simulink model "DR18E_Testpult"  (R2017a)
settings: Solver=ode1  StartTime=0.0  StopTime=Inf  FixedStep=0.001  RelTol=1e-3
PostLoadFcn:
  | , if any(exist('dsrtsu_mdlpostloadfcn', 'file') == [2, 3, 6]), try dsrtsu_mdlpostloadfcn('Execute', bdroot); catch fprintf('Error in PostLoadFcn (dsrtsu_mdlpostloadfcn) for model "%s":\n %s\n', bdroot, lasterr); end, end,
model workspace: external: MATLAB File C:\Users\DeltaRacing\Documents\dSPACE\MABX_DR18E\Model\DR18E_MABX_Parameter.m (data not in the file)
values from neighbouring files (symbols this model uses):
  am = 1/Ts    (= 1)    [DR18E_MABX_Parameter.m]
  bm = K/Ts    (= 0.05)    [DR18E_MABX_Parameter.m]
  cf = 41350    [DR18E_MABX_Parameter.m]
  cr = 41350    [DR18E_MABX_Parameter.m]
  Derating_HV_Battery_Kapa = 1    [DR18E_MABX_Parameter.m]
  Derating_Start_km = 16    [DR18E_MABX_Parameter.m]
  Drive_Mode = 0    [DR18E_MABX_Parameter.m]
  g = 1    [DR18E_MABX_Parameter.m]
  Gas_Modus = 2    [DR18E_MABX_Parameter.m]
  HV_Power_max = 80    [DR18E_MABX_Parameter.m]
  i_Getriebe = 3.3    [DR18E_MABX_Parameter.m]
  i_Lenkgetriebe = 4.32    [DR18E_MABX_Parameter.m]
  K_SET = 1    [DR18E_MABX_Parameter.m]
  Kapazitaet_HV_Battery_kWh = 6.6    [DR18E_MABX_Parameter.m]
  KW_T_Soll = 37    [DR18E_MABX_Parameter.m]
  lf = 1.2    [DR18E_MABX_Parameter.m]
  lr = 1.15    [DR18E_MABX_Parameter.m]
  m = 310    [DR18E_MABX_Parameter.m]
  M_max = 150    [DR18E_MABX_Parameter.m]
  Power_Limit_onoff = 0    [DR18E_MABX_Parameter.m]
  Reifenradius = 0.2351    [DR18E_MABX_Parameter.m]
  Strecke_Endu_km = 22    [DR18E_MABX_Parameter.m]
  TC_Decr_Gas = 0.00005    (= 5e-05)    [DR18E_MABX_Parameter.m]
  TC_Derivative = 0.4    [DR18E_MABX_Parameter.m]
  TC_Incr_Gas = 0.005    [DR18E_MABX_Parameter.m]
  TC_On = 0    [DR18E_MABX_Parameter.m]
  TC_Relay_Off = 0.065    [DR18E_MABX_Parameter.m]
  TC_Relay_On = 0.07    [DR18E_MABX_Parameter.m]
  TV_Mode = 2    [DR18E_MABX_Parameter.m]
  TV_On = 0    [DR18E_MABX_Parameter.m]
  TV_Override = 1    [DR18E_MABX_Parameter.m]
  y = 0.8    [DR18E_MABX_Parameter.m]
undefined symbols (not defined in the file or in its folder): D, DiscIntNeverNeededParam, I, K_OL, P
libraries: simulink x288, rtican x105, rtiusbflightreclib x40, rti1401lib_dio_type3 x10, simulink_extras x10, rti1401lib_adc_type4 x8, rti1401lib_II_base x7
(part 19 of 28)

== system DR18E_Testpult/Verarbeitung/Temperaturregelung1/ModeSelect1 ==
  Man/Aut Pulse : Inport
  Value Man : Inport  Port=2
  Value Aut : Inport  Port=3
  Constant : Constant  OutDataTypeStr=Inherit: Inherit via back propagation
  Data Type Conversion : DataTypeConversion  OutDataTypeStr=boolean
  J-K Flip-Flop : simulink_extras/Flip Flops/J-K Flip-Flop  initial_condition=0
      settings: SourceProductName=Simulink
  Switch : Switch  Criteria=u2 > Threshold
  Value : Outport
  wires:
  Value Man/1 -> Switch/1
  Value Aut/1 -> Switch/3
  Switch/1 -> Value/1
  Constant/1 -> J-K Flip-Flop/3, J-K Flip-Flop/1
  Man/Aut Pulse/1 -> Data Type Conversion/1
  J-K Flip-Flop/1 -> Switch/2  "Man/!Aut"
  Data Type Conversion/1 -> J-K Flip-Flop/2

== system DR18E_Testpult/Verarbeitung/Temperaturregelung1/ModeSelect2 ==
  Man/Aut Pulse : Inport
  Value Man : Inport  Port=2
  Value Aut : Inport  Port=3
  Constant : Constant  OutDataTypeStr=Inherit: Inherit via back propagation
  Data Type Conversion : DataTypeConversion  OutDataTypeStr=boolean
  J-K Flip-Flop : simulink_extras/Flip Flops/J-K Flip-Flop  initial_condition=0
      settings: SourceProductName=Simulink
  Switch : Switch  Criteria=u2 > Threshold
  Value : Outport
  wires:
  Value Man/1 -> Switch/1
  Value Aut/1 -> Switch/3
  Switch/1 -> Value/1
  Constant/1 -> J-K Flip-Flop/3, J-K Flip-Flop/1
  Man/Aut Pulse/1 -> Data Type Conversion/1
  J-K Flip-Flop/1 -> Switch/2  "Man/!Aut"
  Data Type Conversion/1 -> J-K Flip-Flop/2

== system DR18E_Testpult/Verarbeitung/Temperaturregelung1/PT1 Discrete ==
  u : Inport
  K : Inport  Port=2
  T : Inport  Port=3
  Memory : Memory
  Product : Product
  Product1 : Product
  Subsystem : Subsystem
  Sum : Sum  Inputs=|+-
  Sum1 : Sum  Inputs=|++
  y : Outport
  wires:
  K/1 -> Product/1
  Subsystem/1(T*) -> Product1/1
  u/1 -> Product/2
  Sum/1 -> Product1/2
  Product1/1 -> Sum1/1
  Memory/1 -> Sum1/2, Sum/2
  Sum1/1 -> y/1, Memory/1
  Product/1 -> Sum/1
  T/1 -> Subsystem/1(T)

== system DR18E_Testpult/Verarbeitung/Temperaturregelung1/PT1 Discrete1 ==
  u : Inport
  K : Inport  Port=2
  T : Inport  Port=3
  Memory : Memory
  Product : Product
  Product1 : Product
  Subsystem : Subsystem
  Sum : Sum  Inputs=|+-
  Sum1 : Sum  Inputs=|++
  y : Outport
  wires:
  K/1 -> Product/1
  Subsystem/1(T*) -> Product1/1
  u/1 -> Product/2
  Sum/1 -> Product1/2
  Product1/1 -> Sum1/1
  Memory/1 -> Sum1/2, Sum/2
  Sum1/1 -> y/1, Memory/1
  Product/1 -> Sum/1
  T/1 -> Subsystem/1(T)

== system DR18E_Testpult/Verarbeitung/Umrichter Init Config/Umrichter 1 Init Config ==
  note: TX-Register
  note: TX-Intervallzeit in ms
  Bus Creator : BusCreator  Inputs=8
  Bus Creator1 : BusCreator  Inputs=8
  TXReg1 : Constant  Value=hex2dec('30')  OutDataTypeStr=uint16
  TXReg2 : Constant  Value=hex2dec('27')  OutDataTypeStr=uint16
  TXReg3 : Constant  Value=hex2dec('49')  OutDataTypeStr=uint16
  TXReg4 : Constant  Value=hex2dec('90')  OutDataTypeStr=uint16
  TXReg5 : Constant  Value=hex2dec('40')  OutDataTypeStr=uint16
  TXReg6 : Constant  Value=hex2dec('8F')  OutDataTypeStr=uint16
  TXReg7 : Constant  Value=hex2dec('EB')  OutDataTypeStr=uint16
  TXReg8 : Constant  Value=hex2dec('4A')  OutDataTypeStr=uint16
  TXZeit1 : Constant  Value=127  OutDataTypeStr=uint16
  TXZeit2 : Constant  Value=129  OutDataTypeStr=uint16
  TXZeit3 : Constant  Value=254  OutDataTypeStr=uint16
  TXZeit4 : Constant  Value=113  OutDataTypeStr=uint16
  TXZeit5 : Constant  Value=105  OutDataTypeStr=uint16
  TXZeit6 : Constant  Value=131  OutDataTypeStr=uint16
  TXZeit7 : Constant  Value=254  OutDataTypeStr=uint16
  TXZeit8 : Constant  Value=254  OutDataTypeStr=uint16
  tag scope: U1config_TXRegister=global, U1config_TXZeiten=global
  wires:
  Bus Creator/1 -> [U1config_TXRegister]
  TXReg1/1 -> Bus Creator/1  "Drehzahl Istwert"
  TXReg2/1 -> Bus Creator/2  "Drehmoment Istwert"
  TXReg3/1 -> Bus Creator/3  "Motortemp"
  TXReg4/1 -> Bus Creator/4  "DrehmomentSollwert"
  TXReg5/1 -> Bus Creator/5  "Statusmeldung"
  TXReg6/1 -> Bus Creator/6  "Errormeldung"
  TXReg7/1 -> Bus Creator/7  "U_DC"
  TXReg8/1 -> Bus Creator/8  "InverterTemp"
  Bus Creator1/1 -> [U1config_TXZeiten]
  TXZeit1/1 -> Bus Creator1/1
  TXZeit2/1 -> Bus Creator1/2
  TXZeit3/1 -> Bus Creator1/3
  TXZeit4/1 -> Bus Creator1/4
  TXZeit5/1 -> Bus Creator1/5
  TXZeit6/1 -> Bus Creator1/6
  TXZeit7/1 -> Bus Creator1/7
  TXZeit8/1 -> Bus Creator1/8

== system DR18E_Testpult/Verarbeitung/Umrichter Init Config/Umrichter 2 Init Config ==
  note: TX-Register
  note: TX-Intervallzeit in ms
  Bus Creator : BusCreator  Inputs=8
  Bus Creator1 : BusCreator  Inputs=8
  TXReg1 : Constant  Value=hex2dec('30')  OutDataTypeStr=uint16
  TXReg2 : Constant  Value=hex2dec('27')  OutDataTypeStr=uint16
  TXReg3 : Constant  Value=hex2dec('49')  OutDataTypeStr=uint16
  TXReg4 : Constant  Value=hex2dec('90')  OutDataTypeStr=uint16
  TXReg5 : Constant  Value=hex2dec('40')  OutDataTypeStr=uint16
  TXReg6 : Constant  Value=hex2dec('8F')  OutDataTypeStr=uint16
  TXReg7 : Constant  Value=hex2dec('EB')  OutDataTypeStr=uint16
  TXReg8 : Constant  Value=hex2dec('4A')  OutDataTypeStr=uint16
  TXZeit1 : Constant  Value=127  OutDataTypeStr=uint16
  TXZeit2 : Constant  Value=134  OutDataTypeStr=uint16
  TXZeit3 : Constant  Value=254  OutDataTypeStr=uint16
  TXZeit4 : Constant  Value=109  OutDataTypeStr=uint16
  TXZeit5 : Constant  Value=131  OutDataTypeStr=uint16
  TXZeit6 : Constant  Value=103  OutDataTypeStr=uint16
  TXZeit7 : Constant  Value=254  OutDataTypeStr=uint16
  TXZeit8 : Constant  Value=254  OutDataTypeStr=uint16
  tag scope: U2config_TXRegister=global, U2config_TXZeiten=global
  wires:
  Bus Creator/1 -> [U2config_TXRegister]
  TXReg1/1 -> Bus Creator/1  "Drehzahl Istwert"
  TXReg2/1 -> Bus Creator/2  "Drehmoment Istwert"
  TXReg3/1 -> Bus Creator/3  "Motortemp"
  TXReg4/1 -> Bus Creator/4  "DrehmomentSollwert"
  TXReg5/1 -> Bus Creator/5  "Statusmeldung"
  TXReg6/1 -> Bus Creator/6  "Errormeldung"
  TXReg7/1 -> Bus Creator/7  "U_DC"
  TXReg8/1 -> Bus Creator/8  "InverterTemp"
  Bus Creator1/1 -> [U2config_TXZeiten]
  TXZeit1/1 -> Bus Creator1/1
  TXZeit2/1 -> Bus Creator1/2
  TXZeit3/1 -> Bus Creator1/3
  TXZeit4/1 -> Bus Creator1/4
  TXZeit5/1 -> Bus Creator1/5
  TXZeit6/1 -> Bus Creator1/6
  TXZeit7/1 -> Bus Creator1/7
  TXZeit8/1 -> Bus Creator1/8

== system DR18E_Testpult/Verarbeitung/Vehicle State Machine/FlightRecorder ==
  In1 : Inport
  Data Type Conversion : DataTypeConversion
  Gain : Gain
  USB_FLIGHT_REC_BL1 : rtiusbflightreclib/USB_FLIGHT_REC_BL1  VarName=State  DataType=Single  SampleTime=-1  TLCFileName=rtiusbflightrecwrite  Reserved1=[]  Reserved2=[]  Reserved3=[]  Reserved4=[]  DSProperties=struct('RTI',struct('Version',uint32(3),'BlockType',struct('isSLSource',uint8(0),'isSLSink',uint8(1),'isHWSource',uint8(0),'isHWSink',uint8(0),'isSetup',uint8(0),'isInline',uint8(1),'isNonInline',uint8(0),'isInterrupt',uint8(0),'isChannelwise',uint8(0)),'IOBoardType',{{'DSUSB','FLIGHTREC'}},'UnitType','FLIGHTREC','Identifier','WRITE','DialogType','SL','BlockSet','RTIUSBFLIGHTREC','SlaveProcessor','NONE'))  RTIBlockInterface=struct('InputPortsActive',1,'InputPortsWidth',int32(1),'InputPortsDataType',{{'SS_SINGLE'}},'BlockDisplay',{{['Write to\nUSB Flight Recorder'],'center'}},'IconTransparency','off','InitLevel',3,'BlockName',struct('Token',{{'USB_FLIGHT_REC_BL1'}}),'MaskDescription',['Write input to the Flight Recorder. Recorded data can be referenced by the specified variable.'],'SampleTime',{{-1}})  RTIBlockParameters=struct('VarName',{{'State','OFF',[]}},'DataType',{{'Single','OFF',[]}},'SampleTime',{{-1,'OFF',[]}},'TLCFileName',{{'rtiusbflightrecwrite','OFF',[]}})  RTISFcnParameters=struct('VarName','char','DataType','char','SampleTime','double','TLCFileName','char')  RTIBlockParaDefault=struct('VarName','Var1','DataType','Single','SampleTime',-1,'TLCFileName','rtiusbflightrecwrite')
      settings: SourceProductName=dSPACE RTI USB Flight Rec Blockset
  wires:
  Data Type Conversion/1 -> USB_FLIGHT_REC_BL1/1
  In1/1 -> Gain/1
  Gain/1 -> Data Type Conversion/1

== system DR18E_Testpult/Verarbeitung/Vehicle State Machine/FlightRecorder1 ==
  In1 : Inport
  Data Type Conversion : DataTypeConversion
  Gain : Gain
  USB_FLIGHT_REC_BL1 : rtiusbflightreclib/USB_FLIGHT_REC_BL1  VarName=ErrorNo  DataType=Single  SampleTime=-1  TLCFileName=rtiusbflightrecwrite  Reserved1=[]  Reserved2=[]  Reserved3=[]  Reserved4=[]  DSProperties=struct('RTI',struct('Version',uint32(3),'BlockType',struct('isSLSource',uint8(0),'isSLSink',uint8(1),'isHWSource',uint8(0),'isHWSink',uint8(0),'isSetup',uint8(0),'isInline',uint8(1),'isNonInline',uint8(0),'isInterrupt',uint8(0),'isChannelwise',uint8(0)),'IOBoardType',{{'DSUSB','FLIGHTREC'}},'UnitType','FLIGHTREC','Identifier','WRITE','DialogType','SL','BlockSet','RTIUSBFLIGHTREC','SlaveProcessor','NONE'))  RTIBlockInterface=struct('InputPortsActive',1,'InputPortsWidth',int32(1),'InputPortsDataType',{{'SS_SINGLE'}},'BlockDisplay',{{['Write to\nUSB Flight Recorder'],'center'}},'IconTransparency','off','InitLevel',3,'BlockName',struct('Token',{{'USB_FLIGHT_REC_BL1'}}),'MaskDescription',['Write input to the Flight Recorder. Recorded data can be referenced by the specified variable.'],'SampleTime',{{-1}})  RTIBlockParameters=struct('VarName',{{'ErrorNo','OFF',[]}},'DataType',{{'Single','OFF',[]}},'SampleTime',{{-1,'OFF',[]}},'TLCFileName',{{'rtiusbflightrecwrite','OFF',[]}})  RTISFcnParameters=struct('VarName','char','DataType','char','SampleTime','double','TLCFileName','char')  RTIBlockParaDefault=struct('VarName','Var1','DataType','Single','SampleTime',-1,'TLCFileName','rtiusbflightrecwrite')
      settings: SourceProductName=dSPACE RTI USB Flight Rec Blockset
  wires:
  Data Type Conversion/1 -> USB_FLIGHT_REC_BL1/1
  In1/1 -> Gain/1
  Gain/1 -> Data Type Conversion/1

== system DR18E_Testpult/Ausgabe/Inverter TX/Inverters TXTorque/TorqueMessage ==
  RegID_L_R : Inport
  Value32_L_R : Inport  Port=2
  Demux : Demux  Outputs=2
  Demux1 : Demux  Outputs=2
  U1_RegID : Outport
  U1_Value32 : Outport  Port=2
  U2_RegID : Outport  Port=3
  U2_Value32 : Outport  Port=4
  wires:
  Demux/2 -> U2_Value32/1
  Demux/1 -> U1_Value32/1
  Value32_L_R/1 -> Demux/1
  Demux1/1 -> U1_RegID/1
  Demux1/2 -> U2_RegID/1
  RegID_L_R/1 -> Demux1/1

== system DR18E_Testpult/Ausgabe/Inverter TX/Inverters TXUniversal/TorqueMessage ==
  RegID_L_R : Inport
  Value32_L_R : Inport  Port=2
  Demux : Demux  Outputs=2
  Demux1 : Demux  Outputs=2
  U1_RegID : Outport
  U1_Value32 : Outport  Port=2
  U2_RegID : Outport  Port=3
  U2_Value32 : Outport  Port=4
  wires:
  Demux/2 -> U2_Value32/1
  Demux/1 -> U1_Value32/1
  Value32_L_R/1 -> Demux/1
  Demux1/1 -> U1_RegID/1
  Demux1/2 -> U2_RegID/1
  RegID_L_R/1 -> Demux1/1

== system DR18E_Testpult/Ausgabe/Inverter TX/Inverters TXUniversal/Transmit OK Detection1 ==
  note: This subsystem surveys if the sending of the TX message is successful and if it meets the
      | requirements concerning the regularity of the sending.
      |
      | If for 5 consecutive execution steps the message could not be successfully sent the 'TX Warn'
      | output is set to 1. Also, the message is expected to be sent every 50 ms approximatively. If this
      | condition is not met 5 times consecutively the 'TX Warn' output is set to 1.
  TX status : Inport
  TX delta time : Inport  Port=2
  Delta time limit : Constant  Value=0.055
  Delta time limit exceeded : RelationalOperator  RndMeth=Nearest  InputSameDT=on
  Mem{1..4} (4 alike) : Memory
  OR : Logic  Operator=OR
  Prev. msg. not sent : RelationalOperator  Operator=~=  RndMeth=Nearest  InputSameDT=on
  Prev. msg. sent value : Constant
  Warn : Logic  Inputs=5
  TX Warn : Outport
  wires:
  TX delta time/1 -> Delta time limit exceeded/1
  Delta time limit/1 -> Delta time limit exceeded/2
  Prev. msg. sent value/1 -> Prev. msg. not sent/2
  TX status/1 -> Prev. msg. not sent/1
  Prev. msg. not sent/1 -> OR/1
  Delta time limit exceeded/1 -> OR/2
  OR/1 -> Mem1/1, Warn/1
  Mem1/1 -> Mem2/1, Warn/2
  Mem2/1 -> Mem3/1, Warn/3
  Mem3/1 -> Mem4/1, Warn/4
  Mem4/1 -> Warn/5
  Warn/1 -> TX Warn/1

== system DR18E_Testpult/Ausgabe/Inverter TX/Inverters TXUniversal/Transmit OK Detection2 ==
  note: This subsystem surveys if the sending of the TX message is successful and if it meets the
      | requirements concerning the regularity of the sending.
      |
      | If for 5 consecutive execution steps the message could not be successfully sent the 'TX Warn'
      | output is set to 1. Also, the message is expected to be sent every 50 ms approximatively. If this
      | condition is not met 5 times consecutively the 'TX Warn' output is set to 1.
  TX status : Inport
  TX delta time : Inport  Port=2
  Delta time limit : Constant  Value=0.055
  Delta time limit exceeded : RelationalOperator  RndMeth=Nearest  InputSameDT=on
  Mem{1..4} (4 alike) : Memory
  OR : Logic  Operator=OR
  Prev. msg. not sent : RelationalOperator  Operator=~=  RndMeth=Nearest  InputSameDT=on
  Prev. msg. sent value : Constant
  Warn : Logic  Inputs=5
  TX Warn : Outport
  wires:
  TX delta time/1 -> Delta time limit exceeded/1
  Delta time limit/1 -> Delta time limit exceeded/2
  Prev. msg. sent value/1 -> Prev. msg. not sent/2
  TX status/1 -> Prev. msg. not sent/1
  Prev. msg. not sent/1 -> OR/1
  Delta time limit exceeded/1 -> OR/2
  OR/1 -> Mem1/1, Warn/1
  Mem1/1 -> Mem2/1, Warn/2
  Mem2/1 -> Mem3/1, Warn/3
  Mem3/1 -> Mem4/1, Warn/4
  Mem4/1 -> Warn/5
  Warn/1 -> TX Warn/1

== system DR18E_Testpult/Ausgabe/Inverter TX/Umrichter Init/Transmit OK Detection ==
  note: This subsystem surveys if the sending of the TX message is successful and if it meets the
      | requirements concerning the regularity of the sending.
      |
      | If for 5 consecutive execution steps the message could not be successfully sent the 'TX Warn'
      | output is set to 1. Also, the message is expected to be sent every 50 ms approximatively. If this
      | condition is not met 5 times consecutively the 'TX Warn' output is set to 1.
  TX status : Inport
  TX delta time : Inport  Port=2
  Delta time limit : Constant  Value=2
  Delta time limit exceeded : RelationalOperator  RndMeth=Nearest  InputSameDT=on
  Mem{1..4} (4 alike) : Memory
  OR : Logic  Operator=OR
  Prev. msg. not sent : RelationalOperator  Operator=~=  RndMeth=Nearest  InputSameDT=on
  Prev. msg. sent value : Constant
  Rate Transition : RateTransition
  Rate Transition1 : RateTransition
  Warn : Logic  Inputs=5
  TX Warn : Outport
  wires:
  TX delta time/1 -> Rate Transition/1
  Delta time limit/1 -> Delta time limit exceeded/2
  Prev. msg. sent value/1 -> Prev. msg. not sent/2
  TX status/1 -> Rate Transition1/1
  Prev. msg. not sent/1 -> OR/1
  Delta time limit exceeded/1 -> OR/2
  OR/1 -> Mem1/1, Warn/1
  Mem1/1 -> Mem2/1, Warn/2
  Mem2/1 -> Mem3/1, Warn/3
  Mem3/1 -> Mem4/1, Warn/4
  Mem4/1 -> Warn/5
  Warn/1 -> TX Warn/1
  Rate Transition/1 -> Delta time limit exceeded/1
  Rate Transition1/1 -> Prev. msg. not sent/1

== system DR18E_Testpult/Ausgabe/Inverter TX/Umrichter Init/Transmit OK Detection1 ==
  note: This subsystem surveys if the sending of the TX message is successful and if it meets the
      | requirements concerning the regularity of the sending.
      |
      | If for 5 consecutive execution steps the message could not be successfully sent the 'TX Warn'
      | output is set to 1. Also, the message is expected to be sent every 50 ms approximatively. If this
      | condition is not met 5 times consecutively the 'TX Warn' output is set to 1.
  TX status : Inport
  TX delta time : Inport  Port=2
  Delta time limit : Constant  Value=2
  Delta time limit exceeded : RelationalOperator  RndMeth=Nearest  InputSameDT=on
  Mem{1..4} (4 alike) : Memory
  OR : Logic  Operator=OR
  Prev. msg. not sent : RelationalOperator  Operator=~=  RndMeth=Nearest  InputSameDT=on
  Prev. msg. sent value : Constant
  Rate Transition : RateTransition
  Rate Transition1 : RateTransition
  Warn : Logic  Inputs=5
  TX Warn : Outport
  wires:
  TX delta time/1 -> Rate Transition/1
  Delta time limit/1 -> Delta time limit exceeded/2
  Prev. msg. sent value/1 -> Prev. msg. not sent/2
  TX status/1 -> Rate Transition1/1
  Prev. msg. not sent/1 -> OR/1
  Delta time limit exceeded/1 -> OR/2
  OR/1 -> Mem1/1, Warn/1
  Mem1/1 -> Mem2/1, Warn/2
  Mem2/1 -> Mem3/1, Warn/3
  Mem3/1 -> Mem4/1, Warn/4
  Mem4/1 -> Warn/5
  Warn/1 -> TX Warn/1
  Rate Transition/1 -> Delta time limit exceeded/1
  Rate Transition1/1 -> Prev. msg. not sent/1

== system DR18E_Testpult/Eingabe Fahrzeug/BMS/RX Timeout Detection2/Subsystem ==
  TXStatus : Inport
  Timeout : Inport  Port=2
  Constant : Constant
  Constant1 : Constant  Value=0
  Constant2 : Constant
  Constant3 : Constant  Value=0
  Delay : Delay  DelayLength=1  InitialCondition=0
  Relational Operator : RelationalOperator  Operator=>  OutDataTypeStr=boolean  RndMeth=Nearest
  Sum : Sum  Inputs=|++
  Switch : Switch  Criteria=u2 > Threshold
  Switch1 : Switch  Criteria=u2 > Threshold
  Rampe : Outport
  RX Timeout Error : Outport  Port=2
  wires:
  TXStatus/1 -> Switch/2
  Delay/1 -> Sum/2
  Constant/1 -> Sum/1
  Sum/1 -> Switch/3
  Switch/1 -> Delay/1, Relational Operator/1, Rampe/1
  Constant1/1 -> Switch/1
  Constant2/1 -> Switch1/1
  Constant3/1 -> Switch1/3
  Switch1/1 -> RX Timeout Error/1
  Relational Operator/1 -> Switch1/2
  Timeout/1 -> Relational Operator/2

== system DR18E_Testpult/Eingabe Fahrzeug/BMS/STK1-5_Temp /RX Timeout Detection1 ==
  RX status : Inport
  Timeout (n Samples) : Inport  Port=2
  Subsystem : Subsystem  TreatAsAtomicUnit=on
  Terminator_4 : Terminator
  RX Timeout Error : Outport
  wires:
  RX status/1 -> Subsystem/1(TXStatus)
  Subsystem/1(Rampe) -> Terminator_4/1
  Subsystem/2(RX Timeout Error) -> RX Timeout Error/1  "RX Timeout"
  Timeout (n Samples)/1 -> Subsystem/2(Timeout)

== system DR18E_Testpult/Eingabe Fahrzeug/BMS/STK1-5_Temp /RX Timeout Detection10 ==
  RX status : Inport
  Timeout (n Samples) : Inport  Port=2
  Subsystem : Subsystem  TreatAsAtomicUnit=on
  Terminator_4 : Terminator
  RX Timeout Error : Outport
  wires:
  RX status/1 -> Subsystem/1(TXStatus)
  Subsystem/1(Rampe) -> Terminator_4/1
  Subsystem/2(RX Timeout Error) -> RX Timeout Error/1  "RX Timeout"
  Timeout (n Samples)/1 -> Subsystem/2(Timeout)

== system DR18E_Testpult/Eingabe Fahrzeug/BMS/STK1-5_Temp /RX Timeout Detection2 ==
  RX status : Inport
  Timeout (n Samples) : Inport  Port=2
  Subsystem : Subsystem  TreatAsAtomicUnit=on
  Terminator_4 : Terminator
  RX Timeout Error : Outport
  wires:
  RX status/1 -> Subsystem/1(TXStatus)
  Subsystem/1(Rampe) -> Terminator_4/1
  Subsystem/2(RX Timeout Error) -> RX Timeout Error/1  "RX Timeout"
  Timeout (n Samples)/1 -> Subsystem/2(Timeout)

== system DR18E_Testpult/Eingabe Fahrzeug/BMS/STK1-5_Temp /RX Timeout Detection3 ==
  RX status : Inport
  Timeout (n Samples) : Inport  Port=2
  Subsystem : Subsystem  TreatAsAtomicUnit=on
  Terminator_4 : Terminator
  RX Timeout Error : Outport
  wires:
  RX status/1 -> Subsystem/1(TXStatus)
  Subsystem/1(Rampe) -> Terminator_4/1
  Subsystem/2(RX Timeout Error) -> RX Timeout Error/1  "RX Timeout"
  Timeout (n Samples)/1 -> Subsystem/2(Timeout)

== system DR18E_Testpult/Eingabe Fahrzeug/BMS/STK1-5_Temp /RX Timeout Detection4 ==
  RX status : Inport
  Timeout (n Samples) : Inport  Port=2
  Subsystem : Subsystem  TreatAsAtomicUnit=on
  Terminator_4 : Terminator
  RX Timeout Error : Outport
  wires:
  RX status/1 -> Subsystem/1(TXStatus)
  Subsystem/1(Rampe) -> Terminator_4/1
  Subsystem/2(RX Timeout Error) -> RX Timeout Error/1  "RX Timeout"
  Timeout (n Samples)/1 -> Subsystem/2(Timeout)

== system DR18E_Testpult/Eingabe Fahrzeug/BMS/STK1-5_Temp /RX Timeout Detection5 ==
  RX status : Inport
  Timeout (n Samples) : Inport  Port=2
  Subsystem : Subsystem  TreatAsAtomicUnit=on
  Terminator_4 : Terminator
  RX Timeout Error : Outport
  wires:
  RX status/1 -> Subsystem/1(TXStatus)
  Subsystem/1(Rampe) -> Terminator_4/1
  Subsystem/2(RX Timeout Error) -> RX Timeout Error/1  "RX Timeout"
  Timeout (n Samples)/1 -> Subsystem/2(Timeout)

== system DR18E_Testpult/Eingabe Fahrzeug/BMS/STK1-5_Temp /RX Timeout Detection6 ==
  RX status : Inport
  Timeout (n Samples) : Inport  Port=2
  Subsystem : Subsystem  TreatAsAtomicUnit=on
  Terminator_4 : Terminator
  RX Timeout Error : Outport
  wires:
  RX status/1 -> Subsystem/1(TXStatus)
  Subsystem/1(Rampe) -> Terminator_4/1
  Subsystem/2(RX Timeout Error) -> RX Timeout Error/1  "RX Timeout"
  Timeout (n Samples)/1 -> Subsystem/2(Timeout)

== system DR18E_Testpult/Eingabe Fahrzeug/BMS/STK1-5_Temp /RX Timeout Detection7 ==
  RX status : Inport
  Timeout (n Samples) : Inport  Port=2
  Subsystem : Subsystem  TreatAsAtomicUnit=on
  Terminator_4 : Terminator
  RX Timeout Error : Outport
  wires:
  RX status/1 -> Subsystem/1(TXStatus)
  Subsystem/1(Rampe) -> Terminator_4/1
  Subsystem/2(RX Timeout Error) -> RX Timeout Error/1  "RX Timeout"
  Timeout (n Samples)/1 -> Subsystem/2(Timeout)

== system DR18E_Testpult/Eingabe Fahrzeug/BMS/STK1-5_Temp /RX Timeout Detection8 ==
  RX status : Inport
  Timeout (n Samples) : Inport  Port=2
  Subsystem : Subsystem  TreatAsAtomicUnit=on
  Terminator_4 : Terminator
  RX Timeout Error : Outport
  wires:
  RX status/1 -> Subsystem/1(TXStatus)
  Subsystem/1(Rampe) -> Terminator_4/1
  Subsystem/2(RX Timeout Error) -> RX Timeout Error/1  "RX Timeout"
  Timeout (n Samples)/1 -> Subsystem/2(Timeout)

== system DR18E_Testpult/Eingabe Fahrzeug/BMS/STK1-5_Temp /RX Timeout Detection9 ==
  RX status : Inport
  Timeout (n Samples) : Inport  Port=2
  Subsystem : Subsystem  TreatAsAtomicUnit=on
  Terminator_4 : Terminator
  RX Timeout Error : Outport
  wires:
  RX status/1 -> Subsystem/1(TXStatus)
  Subsystem/1(Rampe) -> Terminator_4/1
  Subsystem/2(RX Timeout Error) -> RX Timeout Error/1  "RX Timeout"
  Timeout (n Samples)/1 -> Subsystem/2(Timeout)

== system DR18E_Testpult/Eingabe Fahrzeug/BMS/STK6-10_Temp/RX Timeout Detection1 ==
  RX status : Inport
  Timeout (n Samples) : Inport  Port=2
  Subsystem : Subsystem  TreatAsAtomicUnit=on
  Terminator_4 : Terminator
  RX Timeout Error : Outport
  wires:
  RX status/1 -> Subsystem/1(TXStatus)
  Subsystem/1(Rampe) -> Terminator_4/1
  Subsystem/2(RX Timeout Error) -> RX Timeout Error/1  "RX Timeout"
  Timeout (n Samples)/1 -> Subsystem/2(Timeout)

== system DR18E_Testpult/Eingabe Fahrzeug/BMS/STK6-10_Temp/RX Timeout Detection10 ==
  RX status : Inport
  Timeout (n Samples) : Inport  Port=2
  Subsystem : Subsystem  TreatAsAtomicUnit=on
  Terminator_4 : Terminator
  RX Timeout Error : Outport
  wires:
  RX status/1 -> Subsystem/1(TXStatus)
  Subsystem/1(Rampe) -> Terminator_4/1
  Subsystem/2(RX Timeout Error) -> RX Timeout Error/1  "RX Timeout"
  Timeout (n Samples)/1 -> Subsystem/2(Timeout)

== system DR18E_Testpult/Eingabe Fahrzeug/BMS/STK6-10_Temp/RX Timeout Detection2 ==
  RX status : Inport
  Timeout (n Samples) : Inport  Port=2
  Subsystem : Subsystem  TreatAsAtomicUnit=on
  Terminator_4 : Terminator
  RX Timeout Error : Outport
  wires:
  RX status/1 -> Subsystem/1(TXStatus)
  Subsystem/1(Rampe) -> Terminator_4/1
  Subsystem/2(RX Timeout Error) -> RX Timeout Error/1  "RX Timeout"
  Timeout (n Samples)/1 -> Subsystem/2(Timeout)

== system DR18E_Testpult/Eingabe Fahrzeug/BMS/STK6-10_Temp/RX Timeout Detection3 ==
  RX status : Inport
  Timeout (n Samples) : Inport  Port=2
  Subsystem : Subsystem  TreatAsAtomicUnit=on
  Terminator_4 : Terminator
  RX Timeout Error : Outport
  wires:
  RX status/1 -> Subsystem/1(TXStatus)
  Subsystem/1(Rampe) -> Terminator_4/1
  Subsystem/2(RX Timeout Error) -> RX Timeout Error/1  "RX Timeout"
  Timeout (n Samples)/1 -> Subsystem/2(Timeout)

== system DR18E_Testpult/Eingabe Fahrzeug/BMS/STK6-10_Temp/RX Timeout Detection4 ==
  RX status : Inport
  Timeout (n Samples) : Inport  Port=2
  Subsystem : Subsystem  TreatAsAtomicUnit=on
  Terminator_4 : Terminator
  RX Timeout Error : Outport
  wires:
  RX status/1 -> Subsystem/1(TXStatus)
  Subsystem/1(Rampe) -> Terminator_4/1
  Subsystem/2(RX Timeout Error) -> RX Timeout Error/1  "RX Timeout"
  Timeout (n Samples)/1 -> Subsystem/2(Timeout)

== system DR18E_Testpult/Eingabe Fahrzeug/BMS/STK6-10_Temp/RX Timeout Detection5 ==
  RX status : Inport
  Timeout (n Samples) : Inport  Port=2
  Subsystem : Subsystem  TreatAsAtomicUnit=on
  Terminator_4 : Terminator
  RX Timeout Error : Outport
  wires:
  RX status/1 -> Subsystem/1(TXStatus)
  Subsystem/1(Rampe) -> Terminator_4/1
  Subsystem/2(RX Timeout Error) -> RX Timeout Error/1  "RX Timeout"
  Timeout (n Samples)/1 -> Subsystem/2(Timeout)

== system DR18E_Testpult/Eingabe Fahrzeug/BMS/STK6-10_Temp/RX Timeout Detection6 ==
  RX status : Inport
  Timeout (n Samples) : Inport  Port=2
  Subsystem : Subsystem  TreatAsAtomicUnit=on
  Terminator_4 : Terminator
  RX Timeout Error : Outport
  wires:
  RX status/1 -> Subsystem/1(TXStatus)
  Subsystem/1(Rampe) -> Terminator_4/1
  Subsystem/2(RX Timeout Error) -> RX Timeout Error/1  "RX Timeout"
  Timeout (n Samples)/1 -> Subsystem/2(Timeout)

== system DR18E_Testpult/Eingabe Fahrzeug/BMS/STK6-10_Temp/RX Timeout Detection7 ==
  RX status : Inport
  Timeout (n Samples) : Inport  Port=2
  Subsystem : Subsystem  TreatAsAtomicUnit=on
  Terminator_4 : Terminator
  RX Timeout Error : Outport
  wires:
  RX status/1 -> Subsystem/1(TXStatus)
  Subsystem/1(Rampe) -> Terminator_4/1
  Subsystem/2(RX Timeout Error) -> RX Timeout Error/1  "RX Timeout"
  Timeout (n Samples)/1 -> Subsystem/2(Timeout)

== system DR18E_Testpult/Eingabe Fahrzeug/BMS/STK6-10_Temp/RX Timeout Detection8 ==
  RX status : Inport
  Timeout (n Samples) : Inport  Port=2
  Subsystem : Subsystem  TreatAsAtomicUnit=on
  Terminator_4 : Terminator
  RX Timeout Error : Outport
  wires:
  RX status/1 -> Subsystem/1(TXStatus)
  Subsystem/1(Rampe) -> Terminator_4/1
  Subsystem/2(RX Timeout Error) -> RX Timeout Error/1  "RX Timeout"
  Timeout (n Samples)/1 -> Subsystem/2(Timeout)

== system DR18E_Testpult/Eingabe Fahrzeug/BMS/STK6-10_Temp/RX Timeout Detection9 ==
  RX status : Inport
  Timeout (n Samples) : Inport  Port=2
  Subsystem : Subsystem  TreatAsAtomicUnit=on
  Terminator_4 : Terminator
  RX Timeout Error : Outport
  wires:
  RX status/1 -> Subsystem/1(TXStatus)
  Subsystem/1(Rampe) -> Terminator_4/1
  Subsystem/2(RX Timeout Error) -> RX Timeout Error/1  "RX Timeout"
  Timeout (n Samples)/1 -> Subsystem/2(Timeout)

== system DR18E_Testpult/Eingabe Fahrzeug/BMS/Voltage 9-10/Voltage Stack 10 ==
  Timeout[samples] : Inport
  Bus Creator : BusCreator  Inputs=12
  HV_STK10A : rtican/RTICAN Receive (RX)   Reserved1=[]  Reserved2=[]  Reserved3=[]  Reserved4=[]  SfcnMessage=[]  Msg_Struct=[]  BoardTypeNo=[]  BoardNo=[]  ChannelNo=[]  Parameters=[]  DialogFcn=[]  UnitName=[]  Revision=[]  UnitValues=[]  DSProperties=struct('RTI',struct('Version',uint32(5),'BlockType',struct('isSLSource',uint8(1),'isSLSink',uint8(1),'isHWSource',uint8(0),'isHWSink',uint8(0),'isSetup',uint8(0),'isInline',uint8(1),'isNonInline',uint8(0),'isInterrupt',uint8(0),'isChannelwise',uint8(0)),'IOBoardType','RTICAN','UnitType','MESSAGE','Identifier','RX','DialogType','MSVC','BlockSet','RTICAN','SlaveProcessor','CAN'))  RTIBlockInterface=struct('OutputPortsWidth',int32([1 1 1 1 1 1 1]),'OutputPortsActive',[1 1 1 1 1 1 1],'OutputPortsName',{{'Cell_Voltage_109','Cell_Voltage_110','Cell_Voltage_111','Cell_Voltage_112',['RX status'],['RX time'],['RX delta time']}},'OutputPortsDataType',{{'SS_DOUBLE','SS_DOUBLE','SS_DOUBLE','SS_DOUBLE','SS_DOUBLE','SS_DOUBLE','SS_DOUBLE'}},'OutputPortsLabel',{{'Cell_Voltage_109','Cell_Voltage_110','Cell_Voltage_111','Cell_Voltage_112','','',''}},'OutputPortsLabelMode','ON','InputPortsWidth',int32(0),'InputPortsActive',0,'DialogFcn','rtican_message_interface_gui','BlockDisplay',{{'','center'}},'IconTransparency','on','ParameterTunableNames',{{}},'InitLevel',3,'BlockName',struct('Token',{{'HV_STK10A'}}),'SampleTime',{{-1}},'TriggerPort',{{'none'}},'EnablePort',{{'none'}})  RTIBlockParameters=struct('BoardTypeNo',{{1,'OFF',[]}},'BoardNo',{{2,'ON',[1 16]}},'ChannelNo',{{1,'ON',[1 2]}},'Parameters',{{struct('DataFileSupport',struct('DataFileSelectedMaster',1,'DataFileSelectedLocal',1,'DataFileName','c:\users\deltaracing\documents\canoe\dr18e\dbc\dr18e.dbc|','DataFileDate',['16-Feb-2019 13:23:09'],'SelectedFile','..\..\..\canoe\dr18e_test\dr18e\dbc\dr18e.dbc','InterfaceFcn','rtican_dbc_file_parser'),'Options',struct('StatusSelected',1,'TimeSelected',1,'DeltaTimeSelected',1,'BytePortSelected',0,'MessageLengthSelected',0,'TriggerPort',struct('Selected',0,'TriggerType',0),'UserCoding',struct('Selected',0,'InterfaceFile','UserDecodingFile','FcnName','UserDecodeFcn','InportSelected',0,'InportWidth',1,'OutportSelected',0,'OutportWidth',1),'EnablePortSelected',0,'SignalOnPortnameSelected',1,'UseRXService',0),'Message',struct('MsgOnBlocknameSelected',1,'MsgName','HV_STK10A','MsgIdFormat',0,'MsgId',363,'MsgLength',8,'NumSignals',4,'SampleTime',-1,'Signal',struct('SgnName',{'Cell_Voltage_109','Cell_Voltage_110','Cell_Voltage_111','Cell_Voltage_112'},'SgnStartBit',{0,16,32,48},'SgnLength',{16,16,16,16},'ByteLayout',{0,0,0,0},'Factor',{0.001,0.001,0.001,0.001},'Offset',{0,0,0,0},'SgnComment',{'','','',''},'SgnUnit',{'V','V','V','V'},'Min',{0,0,0,0},'Max',{0,0,0,0},'SgnType',{0,0,0,0},'SLDataType',{'SS_DOUBLE','SS_DOUBLE','SS_DOUBLE','SS_DOUBLE'},'DataType',{0,0,0,0},'ModeValue',{-1,-1,-1,-1}),'MsgIdNumFormat',0,'MsgComment',{{''}}),'Version',1.2,'general',struct('isFromLib',0)),'OFF',[]}},'GroupId',{{struct('Group',{{'RTICAN'}},'No',1,'Behavior',{{'NAMECHANGE'}},'BlockType',{{'SINK'}},'NameChangeFlag',0),'OFF',[]}},'SFcnRTICANMessage',{{struct('MsgType','RX','SFcnPortType','Scalar','MsgName','HV_STK10A','MsgIdFormat','STD','MsgId',363,'MsgLength',8,'NumSignals',4,'SampleTime',-1,'Signal',struct('SgnName',{'Cell_Voltage_109','Cell_Voltage_110','Cell_Voltage_111','Cell_Voltage_112'},'SgnStartBit',{0,16,32,48},'SgnLength',{16,16,16,16},'ByteLayout',{['little endian'],['little endian'],['little endian'],['little endian']},'Factor',{0.001,0.001,0.001,0.001},'Offset',{0,0,0,0},'SgnType',{'standard','standard','standard','standard'},'SLDataType',{'SS_DOUBLE','SS_DOUBLE','SS_DOUBLE','SS_DOUBLE'},'DataType',{['unsigned int'],['unsigned int'],['unsigned int'],['unsigned int']},'ModeValue',{-1,-1,-1,-1}),'StatusSelected','yes','TimeSelected','yes','DeltaTimeSelected','yes','BytePortSelected','no','MessageLengthSelected','no','TriggerPort',struct('Selected','no','TriggerType',0),'UserCoding',struct('Selected','no','InterfaceFile','UserDecodingFile','FcnName','UserDecodeFcn','InportSelected','no','InportWidth',1,'OutportSelected','no','OutportWidth',1),'EnablePortSelected','no','UseRXService','no','BoardType','DS1','BoardNo',2,'ControllerNo',1),'OFF',[]}},'TLCFileName',{{'rtican_rx_message','OFF',[]}})  RTISFcnParameters=struct('SFcnRTICANMessage','struct','TLCFileName','char')  RTIBlockParaDefault=struct('BoardTypeNo',4302,'BoardNo',1,'ChannelNo',1,'Parameters',struct('DataFileSupport',struct('DataFileSelectedMaster',0,'DataFileSelectedLocal',0,'DataFileName','','DataFileDate','','SelectedFile',['<no file selected>']),'Options',struct('StatusSelected',1,'TimeSelected',1,'DeltaTimeSelected',1,'BytePortSelected',0,'MessageLengthSelected',0,'TriggerPort',struct('Selected',0,'TriggerType','rising'),'UserCoding',struct('Selected',0,'InterfaceFile','UserDecodingFile','FcnName','UserDecodeFcn','InportSelected',0,'InportWidth',1,'OutportSelected',0,'OutportWidth',1),'EnablePortSelected',0,'SignalOnPortnameSelected',1,'UseRXService',0),'Message',struct('MsgOnBlocknameSelected',0,'MsgName',['RX Message'],'MsgIdFormat',0,'MsgId',100,'MsgLength',8,'NumSignals',1,'SampleTime',-1,'Signal',struct('SgnName',['RX signal'],'SgnStartBit',0,'SgnLength',8,'SgnType',0,'ModeValue',-1,'DataType',0,'SLDataType','SS_DOUBLE','ByteLayout',0,'Factor',1,'Offset',0,'Min',0,'Max',255,'SgnComment',{{}},'SgnUnit',''),'MsgIdNumFormat',0,'MsgComment',{{''}}),'Version',1.2,'general',struct('isFromLib',1)),'GroupId',struct('Group',{{'RTICAN'}},'No',1,'Behavior',{{'NAMECHANGE'}},'BlockType',{{'SINK'}},'NameChangeFlag',0),'SFcnRTICANMessage',struct('MsgType','RX','MsgName',['RX Message'],'MsgIdFormat','STD','MsgId',100,'MsgLength',8,'NumSignals',1,'SampleTime',-1,'Signal',struct('SgnName',['RX signal'],'SgnStartBit',0,'SgnLength',8,'SgnType','standard','ModeValue',-1,'DataType',['unsigned int'],'ByteLayout',['little endian'],'SLDataType','SS_DOUBLE','Factor',1,'Offset',0),'StatusSelected','yes','TimeSelected','yes','DeltaTimeSelected','yes','BytePortSelected','no','MessageLengthSelected','no','EnablePortSelected','no','UserCoding',struct('Selected','no','InterfaceFile','UserDecodingFile','FcnName','UserDecodeFcn','InportSelected','no','InportWidth',1,'OutportSelected','no','OutportWidth',1),'TriggerPort',struct('Selected','no','TriggerType','rising'),'UseRXService','no','BoardType','DS4302','BoardNo',1,'ControllerNo',1,'SFcnPortType','Scalar'),'TLCFileName','rtican_rx_message')
      settings: AttributesFormatString=Group Id: RTICAN1\n  SourceProductName=dSPACE RTI CAN Blockset
  HV_STK10B : rtican/RTICAN Receive (RX)   Reserved1=[]  Reserved2=[]  Reserved3=[]  Reserved4=[]  SfcnMessage=[]  Msg_Struct=[]  BoardTypeNo=[]  BoardNo=[]  ChannelNo=[]  Parameters=[]  DialogFcn=[]  UnitName=[]  Revision=[]  UnitValues=[]  DSProperties=struct('RTI',struct('Version',uint32(5),'BlockType',struct('isSLSource',uint8(1),'isSLSink',uint8(1),'isHWSource',uint8(0),'isHWSink',uint8(0),'isSetup',uint8(0),'isInline',uint8(1),'isNonInline',uint8(0),'isInterrupt',uint8(0),'isChannelwise',uint8(0)),'IOBoardType','RTICAN','UnitType','MESSAGE','Identifier','RX','DialogType','MSVC','BlockSet','RTICAN','SlaveProcessor','CAN'))  RTIBlockInterface=struct('OutputPortsWidth',int32([1 1 1 1 1 1 1]),'OutputPortsActive',[1 1 1 1 1 1 1],'OutputPortsName',{{'Cell_Voltage_113','Cell_Voltage_114','Cell_Voltage_115','Cell_Voltage_116',['RX status'],['RX time'],['RX delta time']}},'OutputPortsDataType',{{'SS_DOUBLE','SS_DOUBLE','SS_DOUBLE','SS_DOUBLE','SS_DOUBLE','SS_DOUBLE','SS_DOUBLE'}},'OutputPortsLabel',{{'Cell_Voltage_113','Cell_Voltage_114','Cell_Voltage_115','Cell_Voltage_116','','',''}},'OutputPortsLabelMode','ON','InputPortsWidth',int32(0),'InputPortsActive',0,'DialogFcn','rtican_message_interface_gui','BlockDisplay',{{'','center'}},'IconTransparency','on','ParameterTunableNames',{{}},'InitLevel',3,'BlockName',struct('Token',{{'HV_STK10B'}}),'SampleTime',{{-1}},'TriggerPort',{{'none'}},'EnablePort',{{'none'}})  RTIBlockParameters=struct('BoardTypeNo',{{1,'OFF',[]}},'BoardNo',{{2,'ON',[1 16]}},'ChannelNo',{{1,'ON',[1 2]}},'Parameters',{{struct('DataFileSupport',struct('DataFileSelectedMaster',1,'DataFileSelectedLocal',1,'DataFileName','c:\users\deltaracing\documents\canoe\dr18e\dbc\dr18e.dbc|','DataFileDate',['16-Feb-2019 13:23:09'],'SelectedFile','..\..\..\canoe\dr18e_test\dr18e\dbc\dr18e.dbc','InterfaceFcn','rtican_dbc_file_parser'),'Options',struct('StatusSelected',1,'TimeSelected',1,'DeltaTimeSelected',1,'BytePortSelected',0,'MessageLengthSelected',0,'TriggerPort',struct('Selected',0,'TriggerType',0),'UserCoding',struct('Selected',0,'InterfaceFile','UserDecodingFile','FcnName','UserDecodeFcn','InportSelected',0,'InportWidth',1,'OutportSelected',0,'OutportWidth',1),'EnablePortSelected',0,'SignalOnPortnameSelected',1,'UseRXService',0),'Message',struct('MsgOnBlocknameSelected',1,'MsgName','HV_STK10B','MsgIdFormat',0,'MsgId',364,'MsgLength',8,'NumSignals',4,'SampleTime',-1,'Signal',struct('SgnName',{'Cell_Voltage_113','Cell_Voltage_114','Cell_Voltage_115','Cell_Voltage_116'},'SgnStartBit',{0,16,32,48},'SgnLength',{16,16,16,16},'ByteLayout',{0,0,0,0},'Factor',{0.001,0.001,0.001,0.001},'Offset',{0,0,0,0},'SgnComment',{'','','',''},'SgnUnit',{'V','V','V','V'},'Min',{0,0,0,0},'Max',{0,0,0,0},'SgnType',{0,0,0,0},'SLDataType',{'SS_DOUBLE','SS_DOUBLE','SS_DOUBLE','SS_DOUBLE'},'DataType',{0,0,0,0},'ModeValue',{-1,-1,-1,-1}),'MsgIdNumFormat',0,'MsgComment',{{''}}),'Version',1.2,'general',struct('isFromLib',0)),'OFF',[]}},'GroupId',{{struct('Group',{{'RTICAN'}},'No',1,'Behavior',{{'NAMECHANGE'}},'BlockType',{{'SINK'}},'NameChangeFlag',0),'OFF',[]}},'SFcnRTICANMessage',{{struct('MsgType','RX','SFcnPortType','Scalar','MsgName','HV_STK10B','MsgIdFormat','STD','MsgId',364,'MsgLength',8,'NumSignals',4,'SampleTime',-1,'Signal',struct('SgnName',{'Cell_Voltage_113','Cell_Voltage_114','Cell_Voltage_115','Cell_Voltage_116'},'SgnStartBit',{0,16,32,48},'SgnLength',{16,16,16,16},'ByteLayout',{['little endian'],['little endian'],['little endian'],['little endian']},'Factor',{0.001,0.001,0.001,0.001},'Offset',{0,0,0,0},'SgnType',{'standard','standard','standard','standard'},'SLDataType',{'SS_DOUBLE','SS_DOUBLE','SS_DOUBLE','SS_DOUBLE'},'DataType',{['unsigned int'],['unsigned int'],['unsigned int'],['unsigned int']},'ModeValue',{-1,-1,-1,-1}),'StatusSelected','yes','TimeSelected','yes','DeltaTimeSelected','yes','BytePortSelected','no','MessageLengthSelected','no','TriggerPort',struct('Selected','no','TriggerType',0),'UserCoding',struct('Selected','no','InterfaceFile','UserDecodingFile','FcnName','UserDecodeFcn','InportSelected','no','InportWidth',1,'OutportSelected','no','OutportWidth',1),'EnablePortSelected','no','UseRXService','no','BoardType','DS1','BoardNo',2,'ControllerNo',1),'OFF',[]}},'TLCFileName',{{'rtican_rx_message','OFF',[]}})  RTISFcnParameters=struct('SFcnRTICANMessage','struct','TLCFileName','char')  RTIBlockParaDefault=struct('BoardTypeNo',4302,'BoardNo',1,'ChannelNo',1,'Parameters',struct('DataFileSupport',struct('DataFileSelectedMaster',0,'DataFileSelectedLocal',0,'DataFileName','','DataFileDate','','SelectedFile',['<no file selected>']),'Options',struct('StatusSelected',1,'TimeSelected',1,'DeltaTimeSelected',1,'BytePortSelected',0,'MessageLengthSelected',0,'TriggerPort',struct('Selected',0,'TriggerType','rising'),'UserCoding',struct('Selected',0,'InterfaceFile','UserDecodingFile','FcnName','UserDecodeFcn','InportSelected',0,'InportWidth',1,'OutportSelected',0,'OutportWidth',1),'EnablePortSelected',0,'SignalOnPortnameSelected',1,'UseRXService',0),'Message',struct('MsgOnBlocknameSelected',0,'MsgName',['RX Message'],'MsgIdFormat',0,'MsgId',100,'MsgLength',8,'NumSignals',1,'SampleTime',-1,'Signal',struct('SgnName',['RX signal'],'SgnStartBit',0,'SgnLength',8,'SgnType',0,'ModeValue',-1,'DataType',0,'SLDataType','SS_DOUBLE','ByteLayout',0,'Factor',1,'Offset',0,'Min',0,'Max',255,'SgnComment',{{}},'SgnUnit',''),'MsgIdNumFormat',0,'MsgComment',{{''}}),'Version',1.2,'general',struct('isFromLib',1)),'GroupId',struct('Group',{{'RTICAN'}},'No',1,'Behavior',{{'NAMECHANGE'}},'BlockType',{{'SINK'}},'NameChangeFlag',0),'SFcnRTICANMessage',struct('MsgType','RX','MsgName',['RX Message'],'MsgIdFormat','STD','MsgId',100,'MsgLength',8,'NumSignals',1,'SampleTime',-1,'Signal',struct('SgnName',['RX signal'],'SgnStartBit',0,'SgnLength',8,'SgnType','standard','ModeValue',-1,'DataType',['unsigned int'],'ByteLayout',['little endian'],'SLDataType','SS_DOUBLE','Factor',1,'Offset',0),'StatusSelected','yes','TimeSelected','yes','DeltaTimeSelected','yes','BytePortSelected','no','MessageLengthSelected','no','EnablePortSelected','no','UserCoding',struct('Selected','no','InterfaceFile','UserDecodingFile','FcnName','UserDecodeFcn','InportSelected','no','InportWidth',1,'OutportSelected','no','OutportWidth',1),'TriggerPort',struct('Selected','no','TriggerType','rising'),'UseRXService','no','BoardType','DS4302','BoardNo',1,'ControllerNo',1,'SFcnPortType','Scalar'),'TLCFileName','rtican_rx_message')
      settings: AttributesFormatString=Group Id: RTICAN1\n  SourceProductName=dSPACE RTI CAN Blockset
  HV_STK10C : rtican/RTICAN Receive (RX)   Reserved1=[]  Reserved2=[]  Reserved3=[]  Reserved4=[]  SfcnMessage=[]  Msg_Struct=[]  BoardTypeNo=[]  BoardNo=[]  ChannelNo=[]  Parameters=[]  DialogFcn=[]  UnitName=[]  Revision=[]  UnitValues=[]  DSProperties=struct('RTI',struct('Version',uint32(5),'BlockType',struct('isSLSource',uint8(1),'isSLSink',uint8(1),'isHWSource',uint8(0),'isHWSink',uint8(0),'isSetup',uint8(0),'isInline',uint8(1),'isNonInline',uint8(0),'isInterrupt',uint8(0),'isChannelwise',uint8(0)),'IOBoardType','RTICAN','UnitType','MESSAGE','Identifier','RX','DialogType','MSVC','BlockSet','RTICAN','SlaveProcessor','CAN'))  RTIBlockInterface=struct('OutputPortsWidth',int32([1 1 1 1 1 1 1]),'OutputPortsActive',[1 1 1 1 1 1 1],'OutputPortsName',{{'Cell_Voltage_117','Cell_Voltage_118','Cell_Voltage_119','Cell_Voltage_120',['RX status'],['RX time'],['RX delta time']}},'OutputPortsDataType',{{'SS_DOUBLE','SS_DOUBLE','SS_DOUBLE','SS_DOUBLE','SS_DOUBLE','SS_DOUBLE','SS_DOUBLE'}},'OutputPortsLabel',{{'Cell_Voltage_117','Cell_Voltage_118','Cell_Voltage_119','Cell_Voltage_120','','',''}},'OutputPortsLabelMode','ON','InputPortsWidth',int32(0),'InputPortsActive',0,'DialogFcn','rtican_message_interface_gui','BlockDisplay',{{'','center'}},'IconTransparency','on','ParameterTunableNames',{{}},'InitLevel',3,'BlockName',struct('Token',{{'HV_STK10C'}}),'SampleTime',{{-1}},'TriggerPort',{{'none'}},'EnablePort',{{'none'}})  RTIBlockParameters=struct('BoardTypeNo',{{1,'OFF',[]}},'BoardNo',{{2,'ON',[1 16]}},'ChannelNo',{{1,'ON',[1 2]}},'Parameters',{{struct('DataFileSupport',struct('DataFileSelectedMaster',1,'DataFileSelectedLocal',1,'DataFileName','c:\users\deltaracing\documents\canoe\dr18e\dbc\dr18e.dbc|','DataFileDate',['16-Feb-2019 13:23:09'],'SelectedFile','..\..\..\canoe\dr18e_test\dr18e\dbc\dr18e.dbc','InterfaceFcn','rtican_dbc_file_parser'),'Options',struct('StatusSelected',1,'TimeSelected',1,'DeltaTimeSelected',1,'BytePortSelected',0,'MessageLengthSelected',0,'TriggerPort',struct('Selected',0,'TriggerType',0),'UserCoding',struct('Selected',0,'InterfaceFile','UserDecodingFile','FcnName','UserDecodeFcn','InportSelected',0,'InportWidth',1,'OutportSelected',0,'OutportWidth',1),'EnablePortSelected',0,'SignalOnPortnameSelected',1,'UseRXService',0),'Message',struct('MsgOnBlocknameSelected',1,'MsgName','HV_STK10C','MsgIdFormat',0,'MsgId',365,'MsgLength',8,'NumSignals',4,'SampleTime',-1,'Signal',struct('SgnName',{'Cell_Voltage_117','Cell_Voltage_118','Cell_Voltage_119','Cell_Voltage_120'},'SgnStartBit',{0,16,32,48},'SgnLength',{16,16,16,16},'ByteLayout',{0,0,0,0},'Factor',{0.001,0.001,0.001,0.001},'Offset',{0,0,0,0},'SgnComment',{'','','',''},'SgnUnit',{'V','V','V','V'},'Min',{0,0,0,0},'Max',{0,0,0,0},'SgnType',{0,0,0,0},'SLDataType',{'SS_DOUBLE','SS_DOUBLE','SS_DOUBLE','SS_DOUBLE'},'DataType',{0,0,0,0},'ModeValue',{-1,-1,-1,-1}),'MsgIdNumFormat',0,'MsgComment',{{''}}),'Version',1.2,'general',struct('isFromLib',0)),'OFF',[]}},'GroupId',{{struct('Group',{{'RTICAN'}},'No',1,'Behavior',{{'NAMECHANGE'}},'BlockType',{{'SINK'}},'NameChangeFlag',0),'OFF',[]}},'SFcnRTICANMessage',{{struct('MsgType','RX','SFcnPortType','Scalar','MsgName','HV_STK10C','MsgIdFormat','STD','MsgId',365,'MsgLength',8,'NumSignals',4,'SampleTime',-1,'Signal',struct('SgnName',{'Cell_Voltage_117','Cell_Voltage_118','Cell_Voltage_119','Cell_Voltage_120'},'SgnStartBit',{0,16,32,48},'SgnLength',{16,16,16,16},'ByteLayout',{['little endian'],['little endian'],['little endian'],['little endian']},'Factor',{0.001,0.001,0.001,0.001},'Offset',{0,0,0,0},'SgnType',{'standard','standard','standard','standard'},'SLDataType',{'SS_DOUBLE','SS_DOUBLE','SS_DOUBLE','SS_DOUBLE'},'DataType',{['unsigned int'],['unsigned int'],['unsigned int'],['unsigned int']},'ModeValue',{-1,-1,-1,-1}),'StatusSelected','yes','TimeSelected','yes','DeltaTimeSelected','yes','BytePortSelected','no','MessageLengthSelected','no','TriggerPort',struct('Selected','no','TriggerType',0),'UserCoding',struct('Selected','no','InterfaceFile','UserDecodingFile','FcnName','UserDecodeFcn','InportSelected','no','InportWidth',1,'OutportSelected','no','OutportWidth',1),'EnablePortSelected','no','UseRXService','no','BoardType','DS1','BoardNo',2,'ControllerNo',1),'OFF',[]}},'TLCFileName',{{'rtican_rx_message','OFF',[]}})  RTISFcnParameters=struct('SFcnRTICANMessage','struct','TLCFileName','char')  RTIBlockParaDefault=struct('BoardTypeNo',4302,'BoardNo',1,'ChannelNo',1,'Parameters',struct('DataFileSupport',struct('DataFileSelectedMaster',0,'DataFileSelectedLocal',0,'DataFileName','','DataFileDate','','SelectedFile',['<no file selected>']),'Options',struct('StatusSelected',1,'TimeSelected',1,'DeltaTimeSelected',1,'BytePortSelected',0,'MessageLengthSelected',0,'TriggerPort',struct('Selected',0,'TriggerType','rising'),'UserCoding',struct('Selected',0,'InterfaceFile','UserDecodingFile','FcnName','UserDecodeFcn','InportSelected',0,'InportWidth',1,'OutportSelected',0,'OutportWidth',1),'EnablePortSelected',0,'SignalOnPortnameSelected',1,'UseRXService',0),'Message',struct('MsgOnBlocknameSelected',0,'MsgName',['RX Message'],'MsgIdFormat',0,'MsgId',100,'MsgLength',8,'NumSignals',1,'SampleTime',-1,'Signal',struct('SgnName',['RX signal'],'SgnStartBit',0,'SgnLength',8,'SgnType',0,'ModeValue',-1,'DataType',0,'SLDataType','SS_DOUBLE','ByteLayout',0,'Factor',1,'Offset',0,'Min',0,'Max',255,'SgnComment',{{}},'SgnUnit',''),'MsgIdNumFormat',0,'MsgComment',{{''}}),'Version',1.2,'general',struct('isFromLib',1)),'GroupId',struct('Group',{{'RTICAN'}},'No',1,'Behavior',{{'NAMECHANGE'}},'BlockType',{{'SINK'}},'NameChangeFlag',0),'SFcnRTICANMessage',struct('MsgType','RX','MsgName',['RX Message'],'MsgIdFormat','STD','MsgId',100,'MsgLength',8,'NumSignals',1,'SampleTime',-1,'Signal',struct('SgnName',['RX signal'],'SgnStartBit',0,'SgnLength',8,'SgnType','standard','ModeValue',-1,'DataType',['unsigned int'],'ByteLayout',['little endian'],'SLDataType','SS_DOUBLE','Factor',1,'Offset',0),'StatusSelected','yes','TimeSelected','yes','DeltaTimeSelected','yes','BytePortSelected','no','MessageLengthSelected','no','EnablePortSelected','no','UserCoding',struct('Selected','no','InterfaceFile','UserDecodingFile','FcnName','UserDecodeFcn','InportSelected','no','InportWidth',1,'OutportSelected','no','OutportWidth',1),'TriggerPort',struct('Selected','no','TriggerType','rising'),'UseRXService','no','BoardType','DS4302','BoardNo',1,'ControllerNo',1,'SFcnPortType','Scalar'),'TLCFileName','rtican_rx_message')
      settings: AttributesFormatString=Group Id: RTICAN1\n  SourceProductName=dSPACE RTI CAN Blockset
  Logical Operator : Logic  Operator=OR  Inputs=3  AllPortsSameDT=off  OutDataTypeStr=boolean
  RX Timeout Detection : Subsystem
  RX Timeout Detection1 : Subsystem
  RX Timeout Detection2 : Subsystem
  Cell97-108 : Outport
  TimeoutError : Outport  Port=2
  wires:
  HV_STK10B/5 -> RX Timeout Detection/1(RX status)
  HV_STK10C/5 -> RX Timeout Detection2/1(RX status)
  Bus Creator/1 -> Cell97-108/1  "Cell97-108"
  HV_STK10A/5 -> RX Timeout Detection1/1(RX status)
  RX Timeout Detection2/1(RX Timeout Error) -> Logical Operator/3
  RX Timeout Detection/1(RX Timeout Error) -> Logical Operator/2  "RX Timeout Error"
  RX Timeout Detection1/1(RX Timeout Error) -> Logical Operator/1
  Logical Operator/1 -> TimeoutError/1
  Timeout[samples]/1 -> RX Timeout Detection2/2(Timeout (n Samples)), RX Timeout Detection1/2(Timeout (n Samples)), RX Timeout Detection/2(Timeout (n Samples))
  HV_STK10A/1 -> Bus Creator/1  "Cell_Voltage_109"
  HV_STK10A/2 -> Bus Creator/2  "Cell_Voltage_110"
  HV_STK10A/3 -> Bus Creator/3  "Cell_Voltage_111"
  HV_STK10A/4 -> Bus Creator/4  "Cell_Voltage_112"
  HV_STK10B/1 -> Bus Creator/5  "Cell_Voltage_113"
  HV_STK10B/2 -> Bus Creator/6  "Cell_Voltage_114"
  HV_STK10B/3 -> Bus Creator/7  "Cell_Voltage_115"
  HV_STK10B/4 -> Bus Creator/8  "Cell_Voltage_116"
  HV_STK10C/1 -> Bus Creator/9  "Cell_Voltage_117"
  HV_STK10C/2 -> Bus Creator/10  "Cell_Voltage_118"
  HV_STK10C/3 -> Bus Creator/11  "Cell_Voltage_119"
  HV_STK10C/4 -> Bus Creator/12  "Cell_Voltage_120"
